simulink model "Sim2_ImageProcessor_OA"  (R2021b)
settings: Solver=VariableStepAuto  StartTime=0.0  StopTime=Inf  RelTol=1e-3
InitFcn:
  | %run('settingParams.m')
undefined symbols (not defined in the file or in its folder): ArmInitPos, BodyIndexFrame, BodyTrackingID, ColorJointIndices, DepthJointIndices, dt, gray, HandLeftConfidence, HandLeftState, HandRightConfidence, HandRightState, IsBodyTracked, JointPositions, JointTrackingState, limit_range_ANA, limit_range_IMG, none, range_m, relationOfArmCam, strel, translationVector, Twist, videoinput
libraries: robotlib x5, visionmorphops x4, imaqlib x2, visionstatistics x1
settings Model: Creator=shdet  LastModifiedBy=Hibik
settings SolverCC: AlgebraicLoopSolver=TrustRegion
settings DataIOCC: SaveOutput=off  SignalLogging=off  DSMLogging=off  SaveTime=off  ReturnWorkspaceOutputs=off
settings DebuggingCC: PregeneratedLibrarySubsystemCodeDiagnostic=none  SFMachineParentedDataDiag=warning  ArithmeticOperatorsInVariantConditions=warning
settings SFSimCC: SimUseLocalCustomCode=off  CustomCodeUndefinedFunction=UseInterfaceOnly
settings RTWCC: RTWUseLocalCustomCode=off

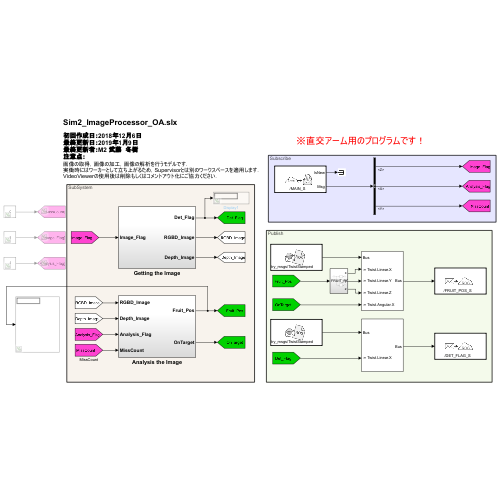
[thumbnail: Simulink's stored preview of the top-level diagram]
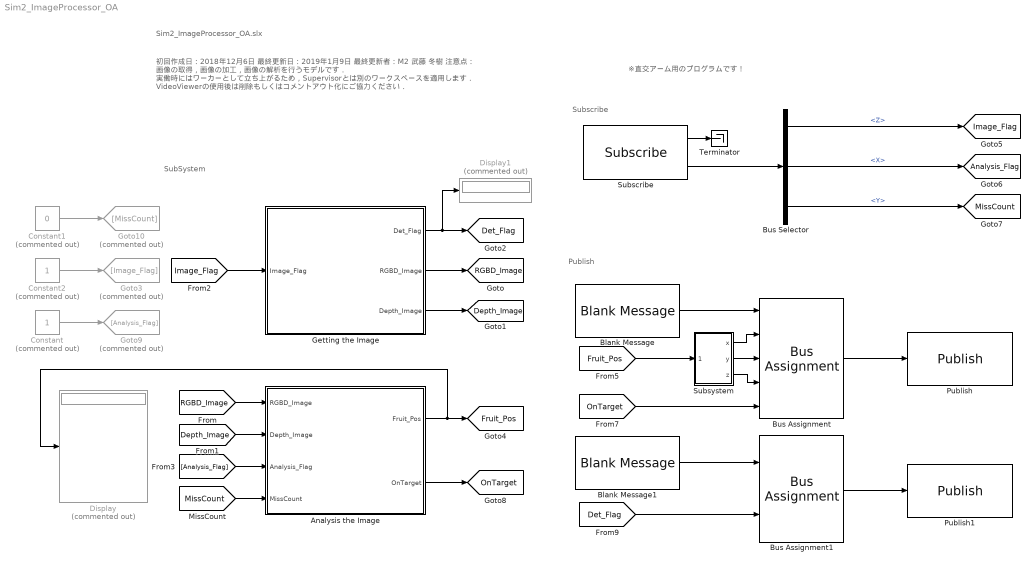
== system Sim2_ImageProcessor_OA ==
  note: Sim2_ImageProcessor_OA.slx
  note: SubSystem
  note: 初回作成日：2018年12月6日
      | 最終更新日：2019年1月9日
      | 最終更新者：M2 武藤 冬樹
      | 注意点：
      | 画像の取得，画像の加工，画像の解析を行うモデルです．
      | 実働時にはワーカーとして立ち上がるため，Supervisorとは別のワークスペースを適用します．
      | VideoViewerの使用後は削除もしくはコメントアウト化にご協力ください．
  note: ※直交アーム用のプログラムです！
  note: Subscribe
  note: Publish
  Analysis the Image : Subsystem
  Blank Message : robotlib/Blank Message  messageClass=Message  entityType=geometry_msgs/TwistStamped  messageType=geometry_msgs/TwistStamped  SampleTime=dt  legacyBusStruct=off
  Blank Message1 : robotlib/Blank Message  messageClass=Message  entityType=geometry_msgs/TwistStamped  messageType=geometry_msgs/TwistStamped  SampleTime=dt  legacyBusStruct=off
  Bus Assignment : BusAssignment  AssignedSignals=Twist.Linear.X,Twist.Linear.Y,Twist.Linear.Z,Twist.Angular.X
  Bus Assignment1 : BusAssignment  AssignedSignals=Twist.Linear.X
  Bus Selector : BusSelector  OutputSignals=Twist.Linear.Z,Twist.Angular.X,Twist.Angular.Y
  Constant : Constant  Commented=on
  Constant1 : Constant  Commented=on  Value=0
  Constant2 : Constant  Commented=on
  Display : Display  Commented=on
  Display1 : Display  Commented=on
  Getting the Image : Subsystem
  Goto10 : Goto  Commented=on  GotoTag=MissCount
  Goto3 : Goto  Commented=on  GotoTag=Image_Flag
  Goto9 : Goto  Commented=on  GotoTag=Analysis_Flag
  Publish : robotlib/Publish  topicSource=Specify your own  topic=/FRUIT_POS_S  messageType=geometry_msgs/TwistStamped  legacyBusStruct=off  messageQueueLength=1
      link override SinkBlock: ROSTopic=FRUIT_POS  ROSMessageType=geometry_msgs/Point  SLBusName=SL_Bus_Sim2_ImageProcesser_geometry_msgs_Point  ModelName=Sim2_ImageProcesser  BlockId=Pub_Sim2_ImageProcesser_396
  Publish1 : robotlib/Publish  topicSource=Specify your own  topic=/DET_FLAG_S  messageType=geometry_msgs/TwistStamped  legacyBusStruct=off  messageQueueLength=1
  Subscribe : robotlib/Subscribe  topicSource=Specify your own  topic=/MAIN_S  messageType=geometry_msgs/TwistStamped  SampleTime=dt  legacyBusStruct=off  messageQueueLength=1
  Subsystem : Subsystem
  Terminator : Terminator
  tag scope: Analysis_Flag=global, Depth_Image=global, Det_Flag=global, Fruit_Pos=global, Image_Flag=global, MissCount=global, OnTarget=global, RGBD_Image=global
  wires:
  Bus Selector/2 -> [Analysis_Flag]  "<X>"
  Subscribe/2 -> Bus Selector/1
  [Fruit_Pos] -> Subsystem/1(FRUIT_POS)
  Blank Message/1 -> Bus Assignment/1
  Blank Message1/1 -> Bus Assignment1/1
  Subscribe/1 -> Terminator/1
  [Det_Flag] -> Bus Assignment1/2
  Bus Assignment1/1 -> Publish1/1
  Subsystem/1(x) -> Bus Assignment/2
  Bus Selector/1 -> [Image_Flag]  "<Z>"
  Subsystem/3(z) -> Bus Assignment/4
  [OnTarget] -> Bus Assignment/5
  Bus Assignment/1 -> Publish/1
  Subsystem/2(y) -> Bus Assignment/3
  Analysis the Image/1(Fruit_Pos) -> Display/1, [Fruit_Pos]
  Analysis the Image/2(OnTarget) -> [OnTarget]
  Getting the Image/2(RGBD_Image) -> [RGBD_Image]
  [RGBD_Image] -> Analysis the Image/1(RGBD_Image)
  [Depth_Image] -> Analysis the Image/2(Depth_Image)
  [Image_Flag] -> Getting the Image/1(Image_Flag)
  [Analysis_Flag] -> Analysis the Image/3(Analysis_Flag)
  Getting the Image/3(Depth_Image) -> [Depth_Image]
  [MissCount] -> Analysis the Image/4(MissCount)
  Getting the Image/1(Det_Flag) -> Display1/1, [Det_Flag]
  Constant/1 -> Goto9/1
  Constant1/1 -> Goto10/1
  Constant2/1 -> Goto3/1
  Bus Selector/3 -> [MissCount]  "<Y>"

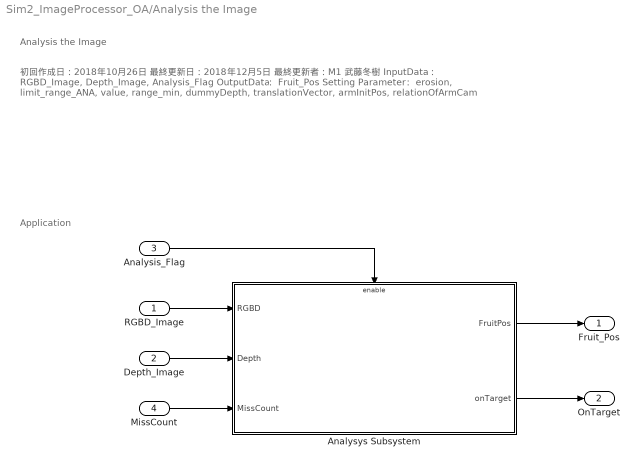
== system Sim2_ImageProcessor_OA/Analysis the Image ==
  note: 初回作成日：2018年10月26日
      | 最終更新日：2018年12月5日
      | 最終更新者：M1 武藤冬樹
      |
      | InputData： RGBD_Image, Depth_Image, Analysis_Flag
      | OutputData： Fruit_Pos
      | Setting Parameter：
      | erosion, limit_range_ANA, value, range_min, dummyDepth, translationVector, armInitPos, relationOfArmCam
  note: Analysis the Image
  note: Application
  RGBD_Image : Inport
  Depth_Image : Inport  Port=2
  Analysis_Flag : Inport  Port=3
  MissCount : Inport  Port=4
  Analysys Subsystem : Subsystem  TreatAsAtomicUnit=on
  Fruit_Pos : Outport  VectorParamsAs1DForOutWhenUnconnected=off
  OnTarget : Outport  Port=2  VectorParamsAs1DForOutWhenUnconnected=off
  wires:
  RGBD_Image/1 -> Analysys Subsystem/1(RGBD)
  Analysis_Flag/1 -> Analysys Subsystem/Enable
  Depth_Image/1 -> Analysys Subsystem/2(Depth)
  Analysys Subsystem/1(FruitPos) -> Fruit_Pos/1
  MissCount/1 -> Analysys Subsystem/3(MissCount)
  Analysys Subsystem/2(onTarget) -> OnTarget/1

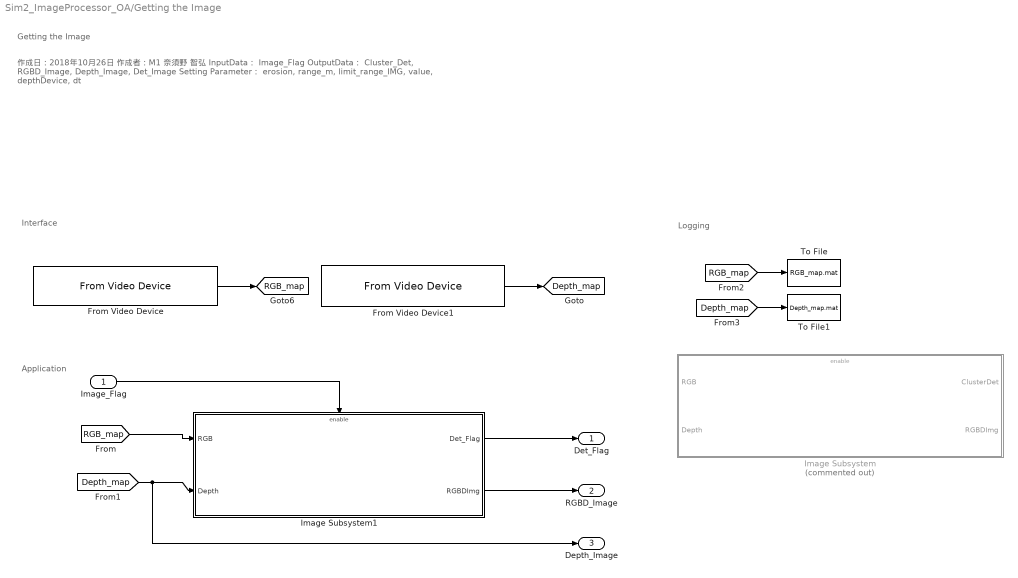
== system Sim2_ImageProcessor_OA/Getting the Image ==
  note: 作成日：2018年10月26日
      | 作成者：M1 奈須野 智弘
      |
      | InputData： Image_Flag
      | OutputData： Cluster_Det, RGBD_Image, Depth_Image, Det_Image
      | Setting Parameter：
      | erosion, range_m, limit_range_IMG, value, depthDevice, dt
  note: Getting the Image
  note: Interface
  note: Application
  note: Logging
  Image_Flag : Inport
  From Video Device : imaqlib/From Video Device  DeviceMenu=(none)  Device=kinect 1 (Kinect V2 Color Sensor)  ObjConstructor=videoinput('kinect', 1)  VideoFormatMenu=(none)  VideoFormat=BGR_1920x1080  VideoSource=Kinect V2 Color Source  ROIPosition=[0 0 1080 1920]  EnableHWTrigger=off  TriggerConfiguration=kinect 1 (Kinect V2 Color Sensor)  SampleTime=0.1  OutputPortsMode=One multidimensional signal  DataType=uint8  CanDoHWTrigger=no  ReturnedColorSpace=rgb  BlockHandle=6.0001  ROIWidth=1920  ROIHeight=1080  ROIColumn=0  ROIRow=0  EngXMLPath=C:\Program Files\MATLAB\R2021b\toolbox\imaq\imaq\private  DevXMLPath=C:\ProgramData\MATLAB\SupportPackages\R2021b\toolbox\imaq\supportpackages\kinectruntime\adaptor\win64  EngLibPath=C:\Program Files\MATLAB\R2021b\toolbox\imaq\imaqblks\imaqmex\win64  ColorSpace=rgb  BayerSensorAlignment=grbg  ImaqMode=off
  From Video Device1 : imaqlib/From Video Device  DeviceMenu=(none)  Device=kinect 2 (Kinect V2 Depth Sensor)  ObjConstructor=videoinput('kinect', 2)  VideoFormatMenu=(none)  VideoFormat=Depth_512x424  VideoSource=Kinect V2 Depth Source  ROIPosition=[0 0 424 512]  EnableHWTrigger=off  TriggerConfiguration=none/none  SampleTime=0.1  OutputPortsMode=One multidimensional signal  DataType=uint16  CanDoHWTrigger=no  ReturnedColorSpace=grayscale  BlockHandle=6.0001  ROIWidth=512  ROIHeight=424  ROIColumn=0  ROIRow=0  EngXMLPath=C:\Program Files\MATLAB\R2021b\toolbox\imaq\imaq\private  DevXMLPath=C:\ProgramData\MATLAB\SupportPackages\R2021b\toolbox\imaq\supportpackages\kinectruntime\adaptor\win64  EngLibPath=C:\Program Files\MATLAB\R2021b\toolbox\imaq\imaqblks\imaqmex\win64  ColorSpace=grayscale  BayerSensorAlignment=grbg  AllMetadata=BodyIndexFrame;BodyTrackingID;ColorJointIndices;DepthJointIndices;HandLeftConfidence;HandLeftState;HandRightConfidence;HandRightState;IsBodyTracked;JointPositions;JointTrackingState  ImaqMode=off
  Image Subsystem : Subsystem  Commented=on  TreatAsAtomicUnit=on
  Image Subsystem1 : Subsystem  TreatAsAtomicUnit=on
  To File : ToFile  Filename=RGB_map.mat  MatrixName=rgb  SaveFormat=Timeseries
  To File1 : ToFile  Filename=Depth_map.mat  MatrixName=depth  SaveFormat=Timeseries
  Det_Flag : Outport  VectorParamsAs1DForOutWhenUnconnected=off
  RGBD_Image : Outport  Port=2  VectorParamsAs1DForOutWhenUnconnected=off
  Depth_Image : Outport  Port=3  VectorParamsAs1DForOutWhenUnconnected=off
  tag scope: Depth_map=global, RGB_map=global
  wires:
  [Depth_map] -> Depth_Image/1, Image Subsystem1/2(Depth)
  [RGB_map] -> Image Subsystem1/1(RGB)
  Image Subsystem1/2(RGBDImg) -> RGBD_Image/1
  Image Subsystem1/1(Det_Flag) -> Det_Flag/1
  From Video Device/1 -> [RGB_map]
  From Video Device1/1 -> [Depth_map]
  Image_Flag/1 -> Image Subsystem1/Enable
  [Depth_map] -> To File1/1
  [RGB_map] -> To File/1

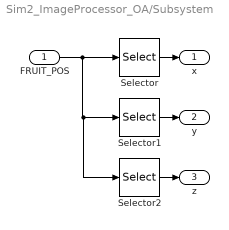
== system Sim2_ImageProcessor_OA/Subsystem ==
  FRUIT_POS : Inport
  Selector : Selector  InputPortWidth=3  IndexOptions=Index vector (dialog)  Indices=1  OutputSizes=1
  Selector1 : Selector  InputPortWidth=3  IndexOptions=Index vector (dialog)  Indices=2  OutputSizes=1
  Selector2 : Selector  InputPortWidth=3  IndexOptions=Index vector (dialog)  Indices=3  OutputSizes=1
  x : Outport  VectorParamsAs1DForOutWhenUnconnected=off
  y : Outport  Port=2  VectorParamsAs1DForOutWhenUnconnected=off
  z : Outport  Port=3  VectorParamsAs1DForOutWhenUnconnected=off
  wires:
  FRUIT_POS/1 -> Selector2/1, Selector1/1, Selector/1
  Selector1/1 -> y/1
  Selector/1 -> x/1
  Selector2/1 -> z/1

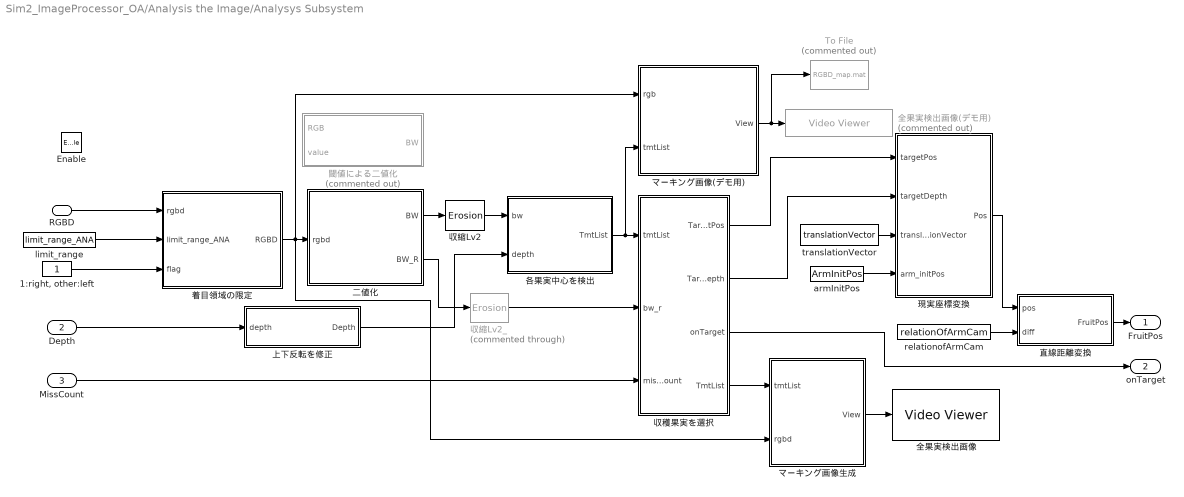
== system Sim2_ImageProcessor_OA/Analysis the Image/Analysys Subsystem ==
  RGBD : Inport
  Depth : Inport  Port=2
  MissCount : Inport  Port=3
  Enable : EnablePort  PropagateVarSize=During execution
  "1:right, other:left" : Constant  SampleTime=dt
  To File : ToFile  Commented=on  Filename=RGBD_map.mat  MatrixName=RGBD  SaveFormat=Timeseries
  armInitPos : Constant  Value=ArmInitPos  VectorParams1D=off  SampleTime=dt
  limit_range : Constant  Value=limit_range_ANA  SampleTime=dt
  relationofArmCam : Constant  Value=relationOfArmCam  VectorParams1D=off  SampleTime=dt
  translationVector : Constant  Value=translationVector  VectorParams1D=off  SampleTime=dt
  マーキング画像(デモ用) : MATLAB Function  TreatAsAtomicUnit=on
  マーキング画像生成 : MATLAB Function  TreatAsAtomicUnit=on
  上下反転を修正 : MATLAB Function  TreatAsAtomicUnit=on
  二値化 : MATLAB Function  TreatAsAtomicUnit=on
  全果実検出画像 : VideoViewer  FigPos=[86 614 418 305]
  全果実検出画像(デモ用) : VideoViewer  Commented=on  colormapValue=gray(256)  FigPos=[717.666666666667 599.333333333333 418 304.666666666667]
  収穫果実を選択 : MATLAB Function  TreatAsAtomicUnit=on
  収縮Lv2 : visionmorphops/Erosion  nhoodsrc=Specify via dialog  strel=strel('disk',4)
      settings: SourceProductBaseCode=VP
  収縮Lv2_ : visionmorphops/Erosion  Commented=through  nhoodsrc=Specify via dialog  strel=strel('disk',2)
      settings: SourceProductBaseCode=VP
  各果実中心を検出 : MATLAB Function  TreatAsAtomicUnit=on
  現実座標変換 : MATLAB Function  TreatAsAtomicUnit=on
  直線距離変換 : MATLAB Function  TreatAsAtomicUnit=on
  着目領域の限定 : MATLAB Function  TreatAsAtomicUnit=on
  閾値による二値化 : MATLAB Function  Commented=on  TreatAsAtomicUnit=on
  FruitPos : Outport  VectorParamsAs1DForOutWhenUnconnected=off
  onTarget : Outport  Port=2  VectorParamsAs1DForOutWhenUnconnected=off
  wires:
  Depth/1 -> 上下反転を修正/1(depth)
  limit_range/1 -> 着目領域の限定/2(limit_range_ANA)
  "1:right, other:left"/1 -> 着目領域の限定/3(flag)
  relationofArmCam/1 -> 直線距離変換/2(diff)
  RGBD/1 -> 着目領域の限定/1(rgbd)
  着目領域の限定/1(RGBD) -> マーキング画像(デモ用)/1(rgb), マーキング画像生成/2(rgbd), 二値化/1(rgbd)
  二値化/1(BW) -> 収縮Lv2/1
  収縮Lv2/1 -> 各果実中心を検出/1(bw)
  各果実中心を検出/1(TmtList) -> マーキング画像(デモ用)/2(tmtList), 収穫果実を選択/1(tmtList)
  収穫果実を選択/2(TargetDepth) -> 現実座標変換/2(targetDepth)
  収穫果実を選択/1(TargetPos) -> 現実座標変換/1(targetPos)
  収穫果実を選択/3(onTarget) -> onTarget/1
  直線距離変換/1(FruitPos) -> FruitPos/1
  上下反転を修正/1(Depth) -> 各果実中心を検出/2(depth)
  armInitPos/1 -> 現実座標変換/4(arm_initPos)
  現実座標変換/1(Pos) -> 直線距離変換/1(pos)
  二値化/2(BW_R) -> 収縮Lv2_/1
  MissCount/1 -> 収穫果実を選択/3(missCount)
  translationVector/1 -> 現実座標変換/3(translationVector)
  収穫果実を選択/4(TmtList) -> マーキング画像生成/1(tmtList)
  マーキング画像生成/1(View) -> 全果実検出画像/1
  マーキング画像(デモ用)/1(View) -> To File/1, 全果実検出画像(デモ用)/1
  収縮Lv2_/1 -> 収穫果実を選択/2(bw_r)

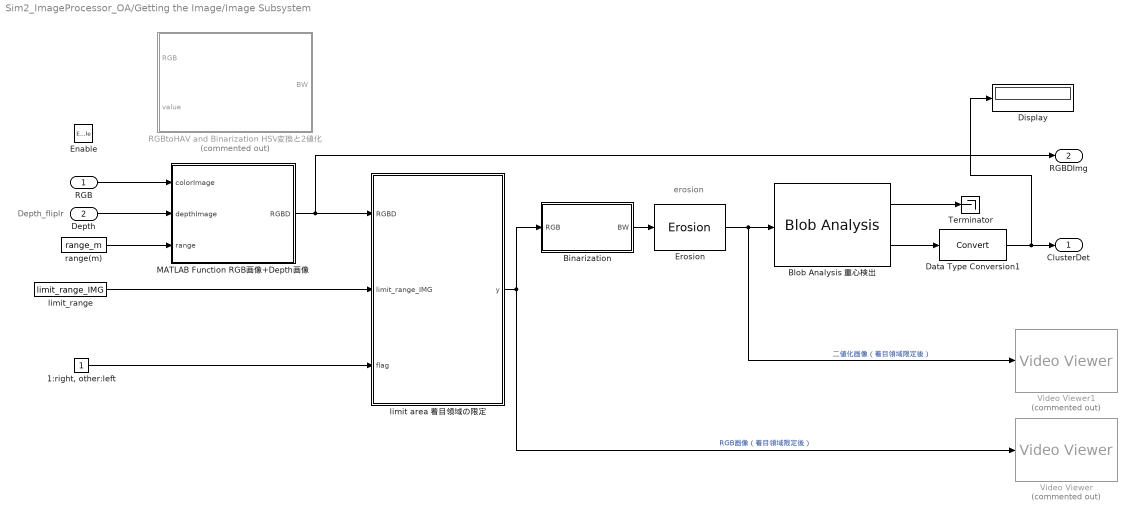
== system Sim2_ImageProcessor_OA/Getting the Image/Image Subsystem ==
  note: Depth_fliplr
  note: erosion
  RGB : Inport
  Depth : Inport  Port=2
  Enable : EnablePort  StatesWhenEnabling=reset
  "1:right, other:left" : Constant  SampleTime=dt
  Binarization : MATLAB Function  TreatAsAtomicUnit=on
  Blob Analysis 重心検出 : visionstatistics/Blob Analysis  Tag=vipblks_row_conv  area=off  centroid=on  bBox=off  majorAxis=off  minorAxis=off  angle=off  eccentricity=off  equivDiameterSq=off  extent=off  perimeter=off  outDT=single  conn=8  isLabel=off  maxBlobs=1  warnIfNumBlobsExceeded=on  isCount=on  useMinArea=off  minArea=3000  useMaxArea=off  maxArea=76800  excludeBorderBlob=off  isOutVarDim=off  isFill=on  fillValues=-1  roundingMode=Floor  overflowMode=off  prodOutputMode=Binary point scaling  prodOutputWordLength=32  prodOutputFracLength=16  prodOutputSlope=2^-16  accumMode=Binary point scaling  accumWordLength=32  accumFracLength=0  accumSlope=2^0  outputMode=Binary point scaling  outputWordLength=32  outputFracLength=16  outputSlope=2^-16  memorySlope=2^-16  firstCoeffMode=Binary point scaling  firstCoeffWordLength=16  firstCoeffFracLength=14  firstCoeffSlope=2^-14  secondCoeffMode=Binary point scaling  secondCoeffWordLength=32  secondCoeffFracLength=16  secondCoeffSlope=2^-16
  Data Type Conversion1 : DataTypeConversion
  Display : Display
  Erosion : visionmorphops/Erosion  nhoodsrc=Specify via dialog  strel=strel('disk',2)
      settings: SourceProductBaseCode=VP
  MATLAB Function RGB画像+Depth画像 : MATLAB Function  TreatAsAtomicUnit=on
  RGBtoHAV and Binarization HSV変換と2値化 : MATLAB Function  Commented=on  TreatAsAtomicUnit=on
  Terminator : Terminator
  Video Viewer : VideoViewer  Commented=on  colormapValue=gray(256)  FigPos=[641.666666666667 337.333333333333 638.666666666667 234.666666666667]
  Video Viewer1 : VideoViewer  Commented=on  colormapValue=gray(256)  FigPos=[641.666666666667 677.333333333333 638.666666666667 234.666666666667]
  limit area 着目領域の限定 : MATLAB Function  TreatAsAtomicUnit=on
  limit_range : Constant  Value=limit_range_IMG  SampleTime=dt
  range(m) : Constant  Value=range_m  SampleTime=dt
  ClusterDet : Outport  OutputWhenDisabled=reset  InitialOutput=0  VectorParamsAs1DForOutWhenUnconnected=off
  RGBDImg : Outport  Port=2  VectorParamsAs1DForOutWhenUnconnected=off
  wires:
  Depth/1 -> MATLAB Function RGB画像+Depth画像/2(depthImage)
  range(m)/1 -> MATLAB Function RGB画像+Depth画像/3(range)
  RGB/1 -> MATLAB Function RGB画像+Depth画像/1(colorImage)
  Blob Analysis 重心検出/2 -> Data Type Conversion1/1
  Blob Analysis 重心検出/1 -> Terminator/1
  limit_range/1 -> limit area 着目領域の限定/2(limit_range_IMG)
  MATLAB Function RGB画像+Depth画像/1(RGBD) -> RGBDImg/1, limit area 着目領域の限定/1(RGBD)
  limit area 着目領域の限定/1(y) -> Binarization/1(RGB), Video Viewer/1  "RGB画像（着目領域限定後）"
  Erosion/1 -> Video Viewer1/1, Blob Analysis 重心検出/1  "二値化画像（着目領域限定後）"
  "1:right, other:left"/1 -> limit area 着目領域の限定/3(flag)
  Binarization/1(BW) -> Erosion/1
  Data Type Conversion1/1 -> Display/1, ClusterDet/1

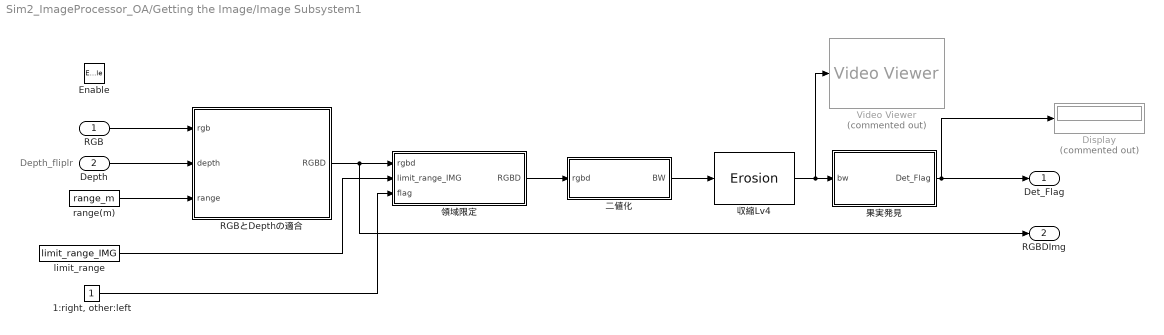
== system Sim2_ImageProcessor_OA/Getting the Image/Image Subsystem1 ==
  note: Depth_fliplr
  RGB : Inport
  Depth : Inport  Port=2
  Enable : EnablePort  StatesWhenEnabling=reset
  "1:right, other:left" : Constant  SampleTime=dt
  Display : Display  Commented=on
  RGBとDepthの適合 : MATLAB Function  TreatAsAtomicUnit=on
  Video Viewer : VideoViewer  Commented=on  colormapValue=gray(256)  FigPos=[14.3333333333333 526 350.666666666667 267.333333333333]
  limit_range : Constant  Value=limit_range_IMG  SampleTime=dt
  range(m) : Constant  Value=range_m  SampleTime=dt
  二値化 : MATLAB Function  TreatAsAtomicUnit=on
  収縮Lv4 : visionmorphops/Erosion  nhoodsrc=Specify via dialog  strel=strel('disk',4)
      settings: SourceProductBaseCode=VP
  果実発見 : MATLAB Function  TreatAsAtomicUnit=on
  領域限定 : MATLAB Function  TreatAsAtomicUnit=on
  Det_Flag : Outport  OutputWhenDisabled=reset  InitialOutput=0  VectorParamsAs1DForOutWhenUnconnected=off
  RGBDImg : Outport  Port=2  VectorParamsAs1DForOutWhenUnconnected=off
  wires:
  Depth/1 -> RGBとDepthの適合/2(depth)
  RGB/1 -> RGBとDepthの適合/1(rgb)
  limit_range/1 -> 領域限定/2(limit_range_IMG)
  RGBとDepthの適合/1(RGBD) -> RGBDImg/1, 領域限定/1(rgbd)
  領域限定/1(RGBD) -> 二値化/1(rgbd)
  収縮Lv4/1 -> Video Viewer/1, 果実発見/1(bw)
  "1:right, other:left"/1 -> 領域限定/3(flag)
  二値化/1(BW) -> 収縮Lv4/1
  果実発見/1(Det_Flag) -> Det_Flag/1, Display/1
  range(m)/1 -> RGBとDepthの適合/3(range)

== matlab function Sim2_ImageProcessor_OA/Getting the Image/Image Subsystem/MATLAB Function RGB画像+Depth画像 ==
  data: colorImage input; RGBD output uint8 size=[424 512 3]; depthImage input; range input
function RGBD  = fcn(colorImage, depthImage, range)

coder.extrinsic('pcfromkinect')
coder.extrinsic('evalin')
coder.extrinsic('getfield')

% depthDevice = imaq.VideoDevice('kinect',2);
device = evalin('base', 'depthDevice');

pc = pcfromkinect(device,depthImage,colorImage, 'depthCentric');
a = single(zeros(424, 512,3));
b = uint8(zeros(424, 512,3));
a = getfield(pc, 'Location');
b = getfield(pc, 'Color');

for i=1:424
   for j=1:512
       if a(i,j,3) < range
           b(i,j,:)=b(i,j,:);
       else
           b(i,j,:)=255;
       end
   end
end

RGBD=b;

% y = single(zeros(424, 512));
% y = fliplr(getfield(pc, 'Location'));
% y = fliplr(y);

== matlab function Sim2_ImageProcessor_OA/Getting the Image/Image Subsystem/RGBtoHAV and Binarization HSV変換と2値化 ==
  data: RGB input; BW output; value input
function BW = createMask(RGB, value)
%createMask  Threshold RGB image using auto-generated code from colorThresholder app.
%  [BW,MASKEDRGBIMAGE] = createMask(RGB) thresholds image RGB using
%  auto-generated code from the colorThresholder App. The colorspace and
%  minimum/maximum values for each channel of the colorspace were set in the
%  App and result in a binary mask BW and a composite image maskedRGBImage,
%  which shows the original RGB image values under the mask BW.

% Auto-generated by colorThresholder app on 12-Apr-2017
%------------------------------------------------------


% Convert RGB image to chosen color space
I = rgb2hsv(RGB);
%%
% H
channel1Min = value(1);
channel1Max = value(2);
% S
channel2Min = value(3);
channel2Max = value(4);
% V
channel3Min = value(5);
channel3Max = value(6);

% Create mask based on chosen histogram thresholds
sliderBW = ( (I(:,:,1) >= channel1Min) | (I(:,:,1) <= channel1Max) ) & ...
    (I(:,:,2) >= channel2Min ) & (I(:,:,2) <= channel2Max) & ...
    (I(:,:,3) >= channel3Min ) & (I(:,:,3) <= channel3Max);
%%
BW = sliderBW;

end

== matlab function Sim2_ImageProcessor_OA/Analysis the Image/Analysys Subsystem/着目領域の限定 ==
  data: rgbd input; RGBD output; limit_range_ANA input; flag input
function RGBD = LimitArea(rgbd, limit_range_ANA, flag)


%{
==============================================================
背景除去をするブロックです。

In: RGB画像（背景除去）、着目領域閾値、アームの取り付け位置に関するフラグ
Out:　RGB画像（背景除去+領域限定）
==============================================================
%}

%===========================
% 上側除去
%===========================
for i=1:limit_range_ANA(1)
    rgbd(i,:,:)=0;
end
%===========================
% 下側除去
%===========================
for i=limit_range_ANA(2):424
    rgbd(i,:,:)=0;
end

%===========================
% 424*512pixel
% 左側除去：flag = 1 : 右側着目
% 右側除去：other    : 左側着目
%===========================
    
if flag==1
    %===========================
    % 左側除去
    %===========================
    for i=1:limit_range_ANA(3)
        rgbd(:,i,:)=0;
    end
    for i=limit_range_ANA(4):512
        rgbd(:,i,:)=0;
    end
else
    %===========================
    % 右側除去
    %===========================
    for i=1:limit_range_ANA(5)
        rgbd(:,i,:)=0;
    end
    for i=limit_range_ANA(6):512
        rgbd(:,i,:)=0;
    end
end

RGBD = rgbd;

== matlab function Sim2_ImageProcessor_OA/Getting the Image/Image Subsystem1/RGBとDepthの適合 ==
  data: rgb input; RGBD output uint8 size=[424 512 3]; depth input; range input
function RGBD = GenarateMainImage(rgb, depth, range)

%{
==============================================================
RGB(1080x1920x3)とDepth(424x512x1)の位置関係を適合
更に奥行き一定以上を背景と見做し除去するブロックです。

In: RGB画像、Depth画像、背景閾値
Out:　RGBD画像（背景除去）
==============================================================
%}

coder.extrinsic('pcfromkinect')
coder.extrinsic('evalin')
coder.extrinsic('getfield')

% depthDevice = imaq.VideoDevice('kinect',2);
device = evalin('base', 'depthDevice');

pc = pcfromkinect(device, depth ,rgb ,'depthCentric');
a = single(zeros(424, 512, 3));
b = uint8(zeros(424, 512, 3));
a = getfield(pc, 'Location');
b = getfield(pc, 'Color');
for i = 1 :424
   for j = 1 :512
       if a(i,j,3) < range
           b(i,j,:) = b(i,j,:);
       else
           b(i,j,:) = 255;
       end
   end
end
RGBD = b;

% y = single(zeros(424, 512));
% y = fliplr(getfield(pc, 'Location'));
% y = fliplr(y);

== matlab function Sim2_ImageProcessor_OA/Getting the Image/Image Subsystem1/果実発見 ==
  data: bw input; Det_Flag output
function Det_Flag = Discovery(bw)

%{
==============================================================
熟した果実の有無を返すブロックです。

In: バイナリ画像
Out:　
==============================================================
%}


h = size(bw, 1);
w = size(bw, 2);
Det_Flag = 0;
for x = 1: w
    for y = 1: h
        if bw(y, x) >= 1
            Det_Flag = 1;
        end
    end
end

== matlab function Sim2_ImageProcessor_OA/Getting the Image/Image Subsystem1/領域限定 ==
  data: rgbd input; RGBD output; limit_range_IMG input; flag input
function RGBD = LimitArea(rgbd, limit_range_IMG, flag)


%{
==============================================================
背景除去をするブロックです。

In: RGB画像（背景除去）、着目領域閾値、アームの取り付け位置に関するフラグ
Out:　RGB画像（背景除去+領域限定）
==============================================================
%}

%===========================
% 上側除去
%===========================
for i=1:limit_range_IMG(1)
    rgbd(i,:,:)=0;
end

%===========================
% 下側除去
%===========================
for i=limit_range_IMG(2):424
    rgbd(i,:,:)=0;
end

%===========================
% 424*512pixel
% 横半分256の半分128±50pixel
% 右側着目：flag = 1 : 左側領域除去：i=78:178
% 左側着目：other    : 右側領域除去：i=334:438
%===========================    
if flag==1
    %===========================
    % 左側除去
    %===========================
    for i=1:limit_range_IMG(3)
        rgbd(:,i,:)=0;
    end
    for i=limit_range_IMG(4):512
        rgbd(:,i,:)=0;
    end
else
    %===========================
    % 右側除去
    %===========================
    for i=1:limit_range_IMG(5)
        rgbd(:,i,:)=0;
    end
    for i=limit_range_IMG(6):512
        rgbd(:,i,:)=0;
    end
end

RGBD = rgbd;

== matlab function Sim2_ImageProcessor_OA/Analysis the Image/Analysys Subsystem/収穫果実を選択 ==
  data: tmtList input; bw_r input; missCount input; TargetPos output; TargetDepth output; onTarget output; TmtList output
function [TargetPos, TargetDepth, onTarget, TmtList] = Selection(tmtList, bw_r, missCount)


%{
==============================================================
収穫する一つのトマトを決めるブロックです。

In: RGB画像（背景除去+領域限定）、トマト情報リスト、バイナリ画像（赤）、連続失敗回数
Out:　XY座標、Depth値、収穫するか否か、マーキング画像

トマト情報リスト
    １：Y座標
    ２：X座標
    ３：Depth値
    ４：評価値
==============================================================
%}


none = 9999;
r = 23;
r2 = r * 2;
listSize = size(tmtList, 1);
%===========================
% ソート（深度昇順）
%===========================
newSize = 0;
for i = 1: listSize
    if tmtList(i, 3) == 0
        tmtList(i, :) = [none, none, none, 0];
    else
        newSize = newSize + 1;
    end
end
tmtList = sortrows(tmtList, 3);

%===========================
% 果実の配置タイプ（房中で上下中央）
%===========================
for i = 1: newSize
    under = 0;
    over = 0;
    for j = 1: newSize
        if i ~= j
            dY = tmtList(i, 1) - tmtList(j, 1);
            dX = tmtList(i, 2) - tmtList(j, 2);
            dZ = tmtList(i, 3) - tmtList(j, 3);
            if abs(dX) < r2 && abs(dY) < r2 && abs(dZ) < 15
                if dY > 0
                    over = 1;
                end
                if dY < 0
                    under = 1;
                end
            end
        end
    end
    %===========================
    % 評価値：(最近傍果実 - 選択果実) - 100 * 配置 + 10000
    %===========================
    tmtList(i, 4) = (tmtList(1, 3) - tmtList(i, 3)) - 100 * over * under + 10000;
end

%===========================
% 高所の果実の評価値を一律減
%===========================
% for i = 1: newSize
%    if tmtList(i, 1) < 200
%       tmtList(i, 4) = tmtList(i, 4) - 1000;
%    end
% end

%===========================
% 未熟トマトの評価値は零
%===========================
for i = 1: newSize
    if bw_r(tmtList(i, 1), tmtList(i, 2)) == 0
        tmtList(i, 4) = 0;
    end
end

%===========================
% ソート（評価値降順）
%===========================
tmtList = sortrows(tmtList, 4, 'descend');

%===========================
% 出力
%===========================
onTarget = 1;
index = missCount + 1;
TargetPos = [tmtList(index, 2), tmtList(index, 1)];
TargetDepth = double(tmtList(index, 3));

if tmtList(index, 4) == 0
    TargetPos = [0, 0];
    onTarget = 0;
end
TmtList = tmtList;

== matlab function Sim2_ImageProcessor_OA/Analysis the Image/Analysys Subsystem/閾値による二値化 ==
  data: RGB input; BW output; value input
function BW = createMask(RGB, value)
%createMask  Threshold RGB image using auto-generated code from colorThresholder app.
%  [BW,MASKEDRGBIMAGE] = createMask(RGB) thresholds image RGB using
%  auto-generated code from the colorThresholder App. The colorspace and
%  minimum/maximum values for each channel of the colorspace were set in the
%  App and result in a binary mask BW and a composite image maskedRGBImage,
%  which shows the original RGB image values under the mask BW.

% Auto-generated by colorThresholder app on 12-Apr-2017
%------------------------------------------------------


% Convert RGB image to chosen color space
I = rgb2hsv(RGB);
%%
% H
channel1Min = value(1);
channel1Max = value(2);
% S
channel2Min = value(3);
channel2Max = value(4);
% V
channel3Min = value(5);
channel3Max = value(6);

% Create mask based on chosen histogram thresholds
sliderBW = ( (I(:,:,1) >= channel1Min) | (I(:,:,1) <= channel1Max) ) & ...
    (I(:,:,2) >= channel2Min ) & (I(:,:,2) <= channel2Max) & ...
    (I(:,:,3) >= channel3Min ) & (I(:,:,3) <= channel3Max);
%%
BW = sliderBW;

end

== matlab function Sim2_ImageProcessor_OA/Analysis the Image/Analysys Subsystem/上下反転を修正 ==
  data: depth input; Depth output
function Depth = Depth_flipr(depth)
    Depth = fliplr(depth);
end

== matlab function Sim2_ImageProcessor_OA/Analysis the Image/Analysys Subsystem/直線距離変換 ==
  data: pos input; FruitPos output size=[1 3]; diff input
function FruitPos = Converter2(pos, diff)


%{
==============================================================
アーム視点の座標に変換するブロックです。

In: 果実の現実座標
Out:　アーム視点の座標
==============================================================
%}


FruitPos = [0, 0, 0];
%===========================
% 直線距離の算出
%Pos(1)=Pos(1)*cos(asin((Pos(2))/Pos(1))) - (90 /pi * asin(Pos(2)/Pos(1))+16)*12; 
%16:16°(関心領域の中心とカメラの角度) 12:距離の補正値(球面だから？距離がずれているのを補正：MP)
%===========================
FruitPos(1) = pos(1) - diff(1); 
%===========================
% y
%===========================
FruitPos(2) = pos(2) - diff(2);
%===========================
% z
%===========================
FruitPos(3) = pos(3) - diff(3);

== matlab function Sim2_ImageProcessor_OA/Getting the Image/Image Subsystem/Binarization ==
  data: RGB input; BW output
function BW = createMask(RGB)
    sigmaI = [85.8997609774271 -39.1553459604252 -38.6963626815188;
        -39.1553459604252 133.189825077682 -61.8149107865788;
        -38.6963626815188 -61.8149107865787 85.4460573367766];

    centroid = [0.377317984497057, 0.51866805610024, 0.304385088726629;
        0.511377845841187 0.682406674784993 0.311679884061617;
        0.258554224598926 0.343365128798657 0.218927575291707;
        0.692867936509784 0.385189498292858 0.222930547134729;
        0.75326742738383 0.783867898551208 0.769989835131869];

    h = size(RGB, 1);
    w = size(RGB, 2);
    BW = false(h, w);
    for x = 1: w
        for y = 1: h
            if RGB(y, x, 1) + RGB(y, x, 2) + RGB(y, x, 3) ~= 0
                r = double(RGB(y, x, 1) * 0.0039216);
                g = double(RGB(y, x, 2) * 0.0039216);
                b = double(RGB(y, x, 3) * 0.0039216);
                minV = 1000000.0;
                bestCluster = -1;
                for i = 1: 5
                    d1 = r - centroid(i, 1);
                    d2 = g - centroid(i, 2);
                    d3 = b - centroid(i, 3);
                    e1 = d1 * sigmaI(1, 1) + d2 * sigmaI(2, 1) + d3 * sigmaI(3, 1);
                    e2 = d1 * sigmaI(1, 2) + d2 * sigmaI(2, 2) + d3 * sigmaI(3, 2);
                    e3 = d1 * sigmaI(1, 3) + d2 * sigmaI(2, 3) + d3 * sigmaI(3, 3);
                    v = (e1 * d1 + e2 * d2 + e3 * d3);
                    if v < minV
                        minV = v;
                        bestCluster = i;
                    end
                end
                %4:fruits, 2:green fruits, 1,3:leaf,steam, 5:others
                if bestCluster == 4
                    BW(y, x) = 1;
                elseif bestCluster == 2
                    BW(y, x) = 0;
                elseif bestCluster == 1 && bestCluster == 3
                    BW(y, x) = 0;
                else
                    BW(y, x) = 0;
                end
            end
        end
    end
end

== matlab function Sim2_ImageProcessor_OA/Analysis the Image/Analysys Subsystem/二値化 ==
  data: rgbd input; BW output; BW_R output
function [BW, BW_R] = Binaryzation(rgbd)


%{
==============================================================
クラスタリングにより二値化をするブロックです。
クラスタリング手法：K-means++法
    K；5
    距離：マハラノビス距離
    元データ：菜園画像（1920*1080）
    判定
    各クラスタインデックスの意味
        4：赤トマト領域
        2；緑トマト領域
        1,3,5：その他

In: RGB画像（背景除去+領域限定）
Out:　バイナリ画像(トマト)、バイナリ画像(熟したトマト)
==============================================================
%}

%===========================
% 逆・分散共分散行列
%===========================
sigmaI = [85.8997609774271 -39.1553459604252 -38.6963626815188;
    -39.1553459604252 133.189825077682 -61.8149107865788;
    -38.6963626815188 -61.8149107865787 85.4460573367766];
%===========================
% クラスタ重心
%===========================
centroid = [0.377317984497057, 0.51866805610024, 0.304385088726629;
    0.511377845841187 0.682406674784993 0.311679884061617;
    0.258554224598926 0.343365128798657 0.218927575291707;
    0.692867936509784 0.385189498292858 0.222930547134729;
    0.75326742738383 0.783867898551208 0.769989835131869];

h = size(rgbd, 1);
w = size(rgbd, 2);
BW = false(h, w);
BW_R = false(h, w);
for x = 1: w
    for y = 1: h
        %===========================
        % 背景or枠外のエリアを除いた各ピクセルは
        % 最近傍のクラスタ重心のインデックスが与えられる
        %===========================
        if rgbd(y, x, 1) + rgbd(y, x, 2) + rgbd(y, x, 3) ~= 0 && rgbd(y, x, 1) + rgbd(y, x, 2) + rgbd(y, x, 3) ~= 765
            r = double(rgbd(y, x, 1) * 0.0039216);
            g = double(rgbd(y, x, 2) * 0.0039216);
            b = double(rgbd(y, x, 3) * 0.0039216);
            minV = 1000000.0;
            bestCluster = -1;
            for i = 1: 5
                d1 = r - centroid(i, 1);
                d2 = g - centroid(i, 2);
                d3 = b - centroid(i, 3);
                e1 = d1 * sigmaI(1, 1) + d2 * sigmaI(2, 1) + d3 * sigmaI(3, 1);
                e2 = d1 * sigmaI(1, 2) + d2 * sigmaI(2, 2) + d3 * sigmaI(3, 2);
                e3 = d1 * sigmaI(1, 3) + d2 * sigmaI(2, 3) + d3 * sigmaI(3, 3);
                v = (e1 * d1 + e2 * d2 + e3 * d3);
                if v < minV
                    minV = v;
                    bestCluster = i;
                end
            end
            %===========================
            % 4：赤トマト領域
            % 2；緑トマト領域
            % 1,3,5：その他
            %===========================
            if bestCluster == 4
                BW(y, x) = 1;
                BW_R(y, x) = 1;
            elseif bestCluster == 2
                BW(y, x) = 1;
                BW_R(y, x) = 0;
            else
                BW(y, x) = 0;
                BW_R(y, x) = 0;
            end
        end
    end
end

== matlab function Sim2_ImageProcessor_OA/Getting the Image/Image Subsystem1/二値化 ==
  data: rgbd input; BW output
function BW = Binaryzation(rgbd)


%{
==============================================================
クラスタリングにより二値化をするブロックです。
クラスタリング手法：K-means++法
    K；5
    距離：マハラノビス距離
    元データ：菜園画像（1920*1080）
    判定
    各クラスタインデックスの意味
        4：赤トマト領域
        2；緑トマト領域
        1,3,5：その他

In: RGB画像（背景除去+領域限定）
Out:　バイナリ画像
==============================================================
%}

%===========================
% 逆・分散共分散行列
%===========================
sigmaI = [85.8997609774271 -39.1553459604252 -38.6963626815188;
    -39.1553459604252 133.189825077682 -61.8149107865788;
    -38.6963626815188 -61.8149107865787 85.4460573367766];
%===========================
% クラスタ重心
%===========================
centroid = [0.377317984497057, 0.51866805610024, 0.304385088726629;
    0.511377845841187 0.682406674784993 0.311679884061617;
    0.258554224598926 0.343365128798657 0.218927575291707;
    0.692867936509784 0.385189498292858 0.222930547134729;
    0.75326742738383 0.783867898551208 0.769989835131869];

h = size(rgbd, 1);
w = size(rgbd, 2);
BW = false(h, w);
for x = 1: w
    for y = 1: h
        %===========================
        % 背景or枠外のエリアを除いた各ピクセルは
        % 最近傍のクラスタ重心のインデックスが与えられる
        %===========================
        if rgbd(y, x, 1) + rgbd(y, x, 2) + rgbd(y, x, 3) ~= 0 && rgbd(y, x, 1) + rgbd(y, x, 2) + rgbd(y, x, 3) ~= 765
            r = double(rgbd(y, x, 1) * 0.0039216);
            g = double(rgbd(y, x, 2) * 0.0039216);
            b = double(rgbd(y, x, 3) * 0.0039216);
            minV = 1000000.0;
            bestCluster = -1;
            for i = 1: 5
                d1 = r - centroid(i, 1);
                d2 = g - centroid(i, 2);
                d3 = b - centroid(i, 3);
                e1 = d1 * sigmaI(1, 1) + d2 * sigmaI(2, 1) + d3 * sigmaI(3, 1);
                e2 = d1 * sigmaI(1, 2) + d2 * sigmaI(2, 2) + d3 * sigmaI(3, 2);
                e3 = d1 * sigmaI(1, 3) + d2 * sigmaI(2, 3) + d3 * sigmaI(3, 3);
                v = (e1 * d1 + e2 * d2 + e3 * d3);
                if v < minV
                    minV = v;
                    bestCluster = i;
                end
            end
            %===========================
            % 4：赤トマト領域
            % 2；緑トマト領域
            % 1,3,5：その他
            %===========================
            if bestCluster == 4
                BW(y, x) = 1;
            elseif bestCluster == 2
                BW(y, x) = 0;
            else
                BW(y, x) = 0;
            end
        end
    end
end

== matlab function Sim2_ImageProcessor_OA/Getting the Image/Image Subsystem/limit area 着目領域の限定 ==
  data: RGBD input; y output; limit_range_IMG input; flag input
function y = fcn(RGBD, limit_range_IMG, flag)

% 上側除去
for i=1:limit_range_IMG(1)
    RGBD(i,:,:)=0;
end
% 下側除去
for i=limit_range_IMG(2):424
    RGBD(i,:,:)=0;
end

% 424*512pixel
% 横半分256の半分128±50pixel
% 右側着目：flag = 1 : 左側領域除去：i=78:178
% 左側着目：other    : 右側領域除去：i=334:438
    
if flag==1
    % 左側除去
    for i=1:limit_range_IMG(3)
        RGBD(:,i,:)=0;
    end
    for i=limit_range_IMG(4):512
        RGBD(:,i,:)=0;
    end
else
    % 右側除去
    for i=1:limit_range_IMG(5)
        RGBD(:,i,:)=0;
    end
    for i=limit_range_IMG(6):512
        RGBD(:,i,:)=0;
    end
end

y=RGBD;

== matlab function Sim2_ImageProcessor_OA/Analysis the Image/Analysys Subsystem/マーキング画像生成 ==
  data: tmtList input; rgbd input; View output
function View = GenerateImage(tmtList, rgbd)


%{
==============================================================
トマトマーカーを含む画像を生成するブロックです。

In: RGB画像（背景除去+領域限定）、トマト情報リスト
Out:　マーキング画像

トマト情報リスト
    １：Y座標
    ２：X座標
    ３：Depth値
    ４：評価値
==============================================================
%}


%===========================
% 描画
% 緑果実　：緑
% 第１候補：橙
% 第２候補：黄
% 以降　　：白
%===========================
listSize = size(tmtList, 1);
View = rgbd;
markR = 6;
[h, w] = size(rgbd);
for i = 1: listSize
    if tmtList(i, 3) ~= 0
        for x = tmtList(i, 2) - markR: tmtList(i, 2) + markR
            for y = tmtList(i, 1) - markR: tmtList(i, 1) + markR
                if x > 0 && y > 0 && x < w && y < h
                    if (x - tmtList(i, 2)) * (x - tmtList(i, 2)) + (y - tmtList(i, 1)) * (y - tmtList(i, 1)) <= markR * markR * 0.5
                        if tmtList(i, 4) == 0
                            View(y, x, :) = [0, 255, 0];
                        elseif i == 1
                            View(y, x, :) = [255, 120, 0];
                        elseif i == 2
                            View(y, x, :) = [255, 255, 0];
                        else
                            View(y, x, :) = [255, 255, 255];
                        end
                    elseif (x - tmtList(i, 2)) * (x - tmtList(i, 2)) + (y - tmtList(i, 1)) * (y - tmtList(i, 1)) <= markR * markR
                            View(y, x, :) = [0, 0, 0];
                    end
                end
            end
        end
    else
        break;
    end
end

== matlab function Sim2_ImageProcessor_OA/Analysis the Image/Analysys Subsystem/マーキング画像(デモ用) ==
  data: rgb input; tmtList input; View output
function View = GenerateImageDemo(rgb, tmtList)


%{
==============================================================
トマトマーカーを含む画像を生成するブロックです。

In: RGB画像（背景除去+領域限定）、トマト情報リスト
Out:　マーキング画像

トマト情報リスト
    １：Y座標
    ２：X座標
    ３：Depth値
    ４：評価値
==============================================================
%}


%===========================
% 描画
%===========================
listSize = size(tmtList, 1);
View = rgb;
markR = 20;
width = 4;
[h, w] = size(rgb);
for i = 1: listSize
    if tmtList(i, 3) ~= 0
        for x = tmtList(i, 2) - markR: tmtList(i, 2) + markR
            for y = tmtList(i, 1) - markR: tmtList(i, 1) + markR
                if x > 0 && y > 0 && x < w && y < h
                    if x - tmtList(i, 2) <= -markR + width || x - tmtList(i, 2) >= markR - width || y - tmtList(i, 1) <= -markR + width || y - tmtList(i, 1) >= markR - width
                        View(y, x, :) = [255, 150, 0];
                    end
                end
            end
        end
    else
        break;
    end
end

== matlab function Sim2_ImageProcessor_OA/Analysis the Image/Analysys Subsystem/現実座標変換 ==
  data: targetPos input; Pos output; targetDepth input; translationVector input; arm_initPos input
function Pos = Converter(targetPos, targetDepth, translationVector ,arm_initPos)


%{
==============================================================
画像座標系(px)を現実座標系(mm)に変換するブロックです。

In: XY座標、Depth値、??、アームの初期位置
Out:　果実の現実座標
==============================================================
%}

coder.extrinsic('evalin', 'pointsToWorld')
Params = evalin('base', 'IRcameraParams');
R = evalin('base', 'R');
% t = evalin('base', 't');
Pos = [0, 0, 0];
if targetPos(2)~=-1 && targetDepth ~= 0
    %ArmX=double(Depthmap(round(u(2)), round(u(1))));
    ArmX=double(targetDepth);
    translationVector(3)=ArmX;
    imagePoints=[targetPos(1), targetPos(2)];

    % 画像座標系(px)を現実座標系(mm)へ
    worldPoints1 = pointsToWorld(Params, R, translationVector, imagePoints);
    % disp(worldPoints1(1));
    % disp(worldPoints1(2));
    ArmY=worldPoints1(1);
    ArmZ=worldPoints1(2);
    %test = round(ArmY) - 80; 
    
    Pos = [ArmX, ArmY, ArmZ];
    Pos(3) = -1 * ArmZ;     % -1をかける
    Pos(2) = Pos(2) -80;    % kinectのずれ補正
else
    Pos = [arm_initPos(1),arm_initPos(2), arm_initPos(3)];
end

== matlab function Sim2_ImageProcessor_OA/Analysis the Image/Analysys Subsystem/各果実中心を検出 ==
  data: bw input; depth input; TmtList output
function TmtList = Detection(bw, depth)


%{
==============================================================
各果実座標をリストで返すブロックです。

径固定球体・逐次検出法を用います。

In: バイナリ画像、Depth画像
Out:　トマト情報リスト


トマト情報リスト
    １：Y座標
    ２：X座標
    ３：Depth値
    ４：評価値
==============================================================
%}


listSize = 30;
none = 9999;
r = 23;
[h, w] = size(bw);
lock = zeros(size(bw));
TmtList = zeros(listSize, 4);
%===========================
% 径固定球体・逐次検出法
%===========================
for count = 1: listSize
    minDepth = uint16(none);
    x = 1;
    y = 1;
    for i = 1: 1: w - 1
        for j = 1: 1: h - 1
            if lock(j, i) == 0 && bw(j, i) == 1 && depth(j, i) ~= 0 && depth(j, i) < minDepth
                minDepth = depth(j, i);
                y = j;
                x = i;
            end
        end
    end
    if minDepth < none
        for i = x - r: x + r
            for j = y - r: y + r
                if (i - x) * (i - x) + (j - y) * (j - y) <= r * r
                    if i > 0 && j > 0 && i < w && j < h
                       lock(j, i) = 1;
                    end
                end
            end
        end
        TmtList(count, :) = [y, x, depth(y, x), 0];
    else
        break;
    end
end
